simulink model "EchtwertVergleich"  (R2021b)
settings: Solver=VariableStepAuto  StartTime=0.0  StopTime=11  RelTol=1e-3
values from neighbouring files (symbols this model uses):
  T = readtable("YawInertiaPendel01.csv")    [ImportTest.m]
settings Model: Creator=tim  LastModifiedBy=tim

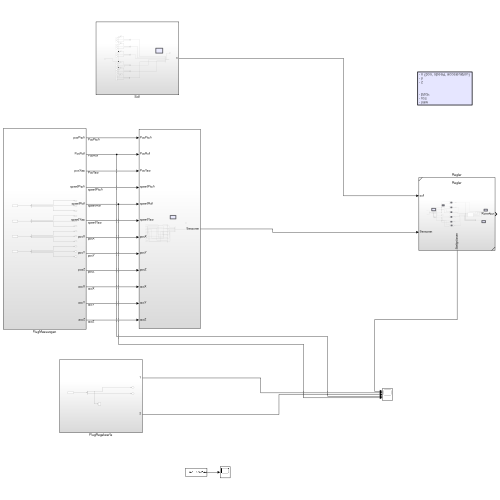
[thumbnail: Simulink's stored preview of the top-level diagram]
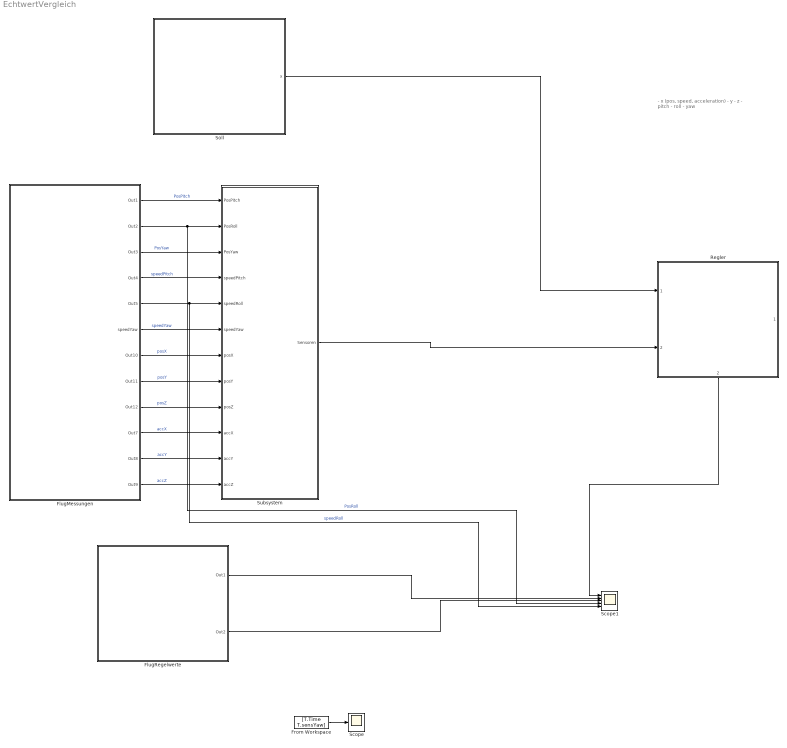
== system EchtwertVergleich ==
  note: - x (pos, speed, acceleration)
      | - y
      | - z
      |
      |
      | - pitch
      | - roll
      | - yaw
  FlugMessungen : Subsystem
  FlugRegelwerte : Subsystem
  From Workspace : FromWorkspace  VariableName=[T.Time T.sensYaw]  SampleTime=T.Time(2) - T.Time(1)  ZeroCross=off  OutputAfterFinalValue=Holding final value
  Regler : Subsystem  VariantControl=Choice  ReferencedSubsystem=Regler
      settings: PortSchema="{\"entries\":[{\"content\":{\"sides\":[{\"content\":{\"connectorIds\":[\"In1\",\"In2\"]},\"type\":\"ConnectorPlacement.EquallySpacedRectSide\",\"uuid\":\"5555f1c3-3fce-4abf-9ec7-ee9d2aa201b7\"},{\"content\":{\"connectorIds\":[\"Out1\"],\"side\":\"RIGHT\"},\"type\":\"ConnectorPlacement.EquallySpacedRectSide\",\"uuid\":\"426c5255-79a7-46e4-b0a4-b934f06d6de9\"},{\"content\":{\"connectorIds\":[],\"side\":\"TOP\"},\"type\":\"ConnectorPlacement.EquallySpacedRectSide\",\"uuid\":\"d67f9dd2-7469-42d8-a750-e83b535a436f\"},{\"content\":{\"connectorIds\":[\"Out2\"],\"side\":\"BOTTOM\"},\"type\":\"ConnectorPlacement.EquallySpacedRectSide\",\"uuid\":\"7dee37cc-875e-40cb-80e0-9d0af31dfaad\"}]},\"type\":\"ConnectorPlacement.EquallySpacedConnector\",\"uuid\":\"ab5c7b53-c15f-43f7-a95d-050bca66474b\"}],\"packageUris\":[\"http://schema.mathworks.com/mf0/Connector/R2020b\"],\"version\":\"1.0\"}"
  Scope : Scope
  Scope1 : Scope  NumInputPorts=5
  Soll : Subsystem
  Subsystem : Subsystem
  wires:
  Soll/1(x) -> Regler/1
  FlugMessungen/1(Out1) -> Subsystem/1(PosPitch)  "PosPitch"
  FlugMessungen/2(Out2) -> Scope1/4, Subsystem/2(PosRoll)  "PosRoll"
  FlugMessungen/3(Out3) -> Subsystem/3(PosYaw)  "PosYaw"
  FlugMessungen/4(Out4) -> Subsystem/4(speedPitch)  "speedPitch"
  FlugMessungen/5(Out5) -> Scope1/5, Subsystem/5(speedRoll)  "speedRoll"
  FlugMessungen/6(speedYaw) -> Subsystem/6(speedYaw)  "speedYaw"
  FlugMessungen/7(Out10) -> Subsystem/7(posX)  "posX"
  FlugMessungen/8(Out11) -> Subsystem/8(posY)  "posY"
  FlugMessungen/9(Out12) -> Subsystem/9(posZ)  "posZ"
  FlugMessungen/10(Out7) -> Subsystem/10(accX)  "accX"
  FlugMessungen/11(Out8) -> Subsystem/11(accY)  "accY"
  FlugMessungen/12(Out9) -> Subsystem/12(accZ)  "accZ"
  Subsystem/1(Sensoren) -> Regler/2
  FlugRegelwerte/1(Out1) -> Scope1/2
  FlugRegelwerte/2(Out2) -> Scope1/3
  Regler/2 -> Scope1/1
  From Workspace/1 -> Scope/1

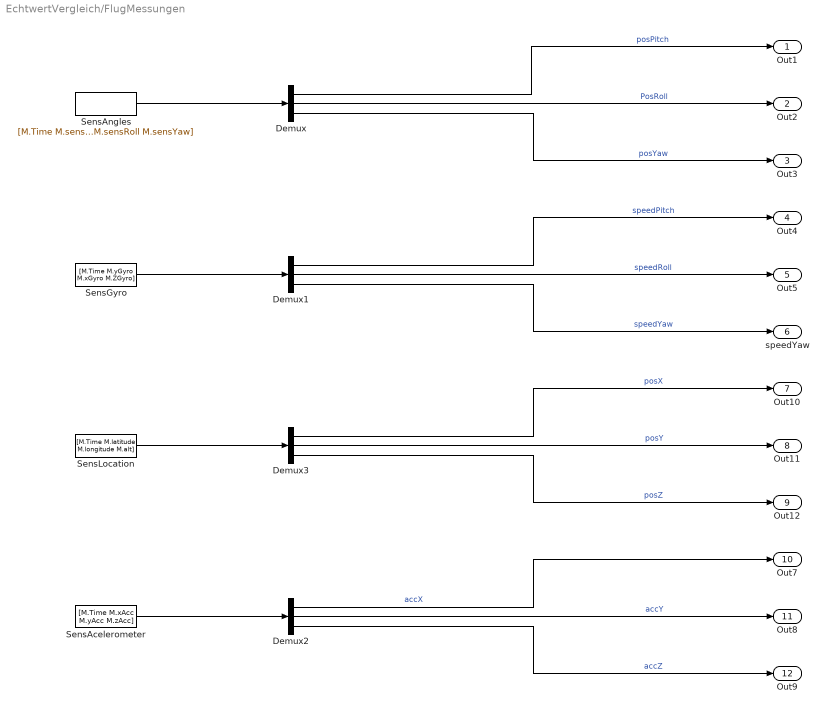
== system EchtwertVergleich/FlugMessungen ==
  Demux{,1..3} (4 alike) : Demux  Outputs=3
  SensAcelerometer : FromWorkspace  VariableName=[M.Time M.xAcc M.yAcc M.zAcc]
  SensAngles : FromWorkspace  VariableName=[M.Time M.sensPitch M.sensRoll M.sensYaw]
  SensGyro : FromWorkspace  VariableName=[M.Time M.yGyro M.xGyro M.ZGyro]
  SensLocation : FromWorkspace  VariableName=[M.Time M.latitude M.longitude M.alt]
  Out1 : Outport
  Out2 : Outport  Port=2
  Out3 : Outport  Port=3
  Out4 : Outport  Port=4
  Out5 : Outport  Port=5
  speedYaw : Outport  Port=6
  Out10 : Outport  Port=7
  Out11 : Outport  Port=8
  Out12 : Outport  Port=9
  Out7 : Outport  Port=10
  Out8 : Outport  Port=11
  Out9 : Outport  Port=12
  wires:
  Demux/1 -> Out1/1  "posPitch"
  Demux/2 -> Out2/1  "PosRoll"
  Demux/3 -> Out3/1  "posYaw"
  Demux1/2 -> Out5/1  "speedRoll"
  Demux2/2 -> Out8/1  "accY"
  Demux2/1 -> Out7/1  "accX"
  Demux2/3 -> Out9/1  "accZ"
  Demux1/3 -> speedYaw/1  "speedYaw"
  Demux1/1 -> Out4/1  "speedPitch"
  Demux3/1 -> Out10/1  "posX"
  Demux3/2 -> Out11/1  "posY"
  Demux3/3 -> Out12/1  "posZ"
  SensAcelerometer/1 -> Demux2/1
  SensLocation/1 -> Demux3/1
  SensAngles/1 -> Demux/1
  SensGyro/1 -> Demux1/1

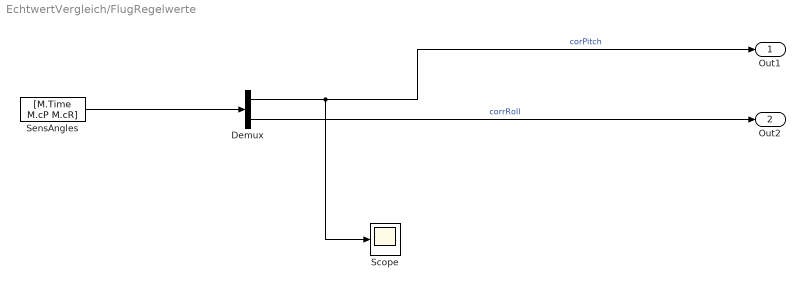
== system EchtwertVergleich/FlugRegelwerte ==
  Demux : Demux  Outputs=2
  Scope : Scope
  SensAngles : FromWorkspace  VariableName=[M.Time M.cP M.cR]  OutputAfterFinalValue=Holding final value
  Out1 : Outport
  Out2 : Outport  Port=2
  wires:
  Demux/2 -> Out2/1  "corrRoll"
  Demux/1 -> Scope/1, Out1/1  "corPitch"
  SensAngles/1 -> Demux/1

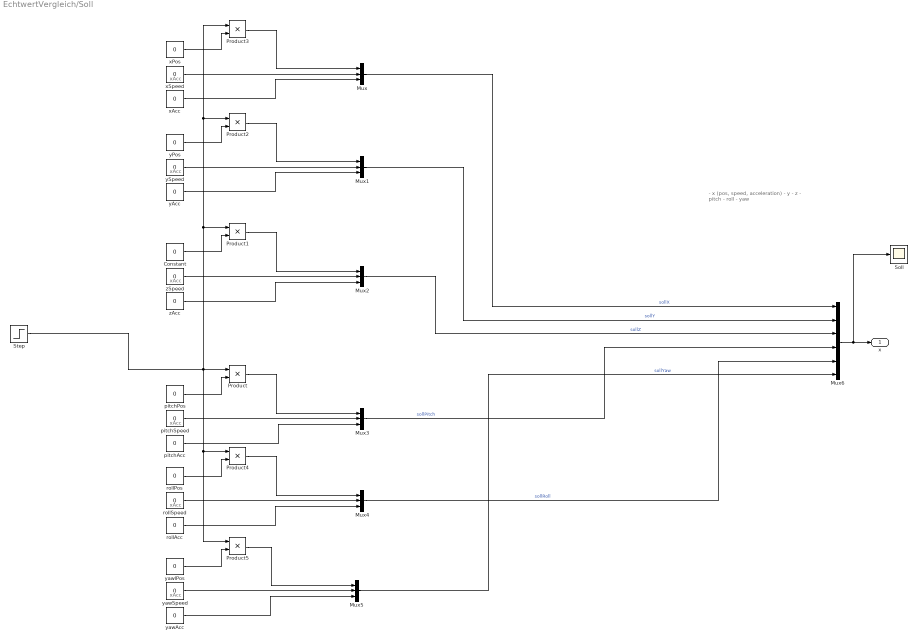
== system EchtwertVergleich/Soll ==
  note: - x (pos, speed, acceleration)
      | - y
      | - z
      |
      |
      | - pitch
      | - roll
      | - yaw
  note: xAcc
  note: xAcc
  note: xAcc
  note: xAcc
  note: xAcc
  note: xAcc
  Constant : Constant  Value=0
  Mux{,1..5} (6 alike) : Mux  Inputs=3
  Mux6 : Mux  Inputs=6
  Product{,1..5} (6 alike) : Product
  Soll : Scope
  Step : Step  SampleTime=0
  pitchAcc : Constant  Value=0
  pitchPos : Constant  Value=0
  pitchSpeed : Constant  Value=0
  rollAcc : Constant  Value=0
  rollPos : Constant  Value=0
  rollSpeed : Constant  Value=0
  xAcc : Constant  Value=0
  xPos : Constant  Value=0
  xSpeed : Constant  Value=0
  yAcc : Constant  Value=0
  yPos : Constant  Value=0
  ySpeed : Constant  Value=0
  yawAcc : Constant  Value=0
  yawSpeed : Constant  Value=0
  yawlPos : Constant  Value=0
  zAcc : Constant  Value=0
  zSpeed : Constant  Value=0
  x : Outport
  wires:
  Mux/1 -> Mux6/1  "sollX"
  Mux1/1 -> Mux6/2  "sollY"
  Mux2/1 -> Mux6/3  "sollZ"
  Mux4/1 -> Mux6/5  "sollRoll"
  Mux5/1 -> Mux6/6  "sollYaw"
  Mux3/1 -> Mux6/4  "sollPitch"
  Mux6/1 -> Soll/1, x/1
  pitchAcc/1 -> Mux3/3
  pitchSpeed/1 -> Mux3/2
  Product/1 -> Mux3/1
  pitchPos/1 -> Product/2
  zAcc/1 -> Mux2/3
  zSpeed/1 -> Mux2/2
  Product1/1 -> Mux2/1
  Constant/1 -> Product1/2
  yAcc/1 -> Mux1/3
  ySpeed/1 -> Mux1/2
  Product2/1 -> Mux1/1
  yPos/1 -> Product2/2
  xAcc/1 -> Mux/3
  xSpeed/1 -> Mux/2
  Product3/1 -> Mux/1
  xPos/1 -> Product3/2
  rollAcc/1 -> Mux4/3
  rollSpeed/1 -> Mux4/2
  Product4/1 -> Mux4/1
  rollPos/1 -> Product4/2
  yawlPos/1 -> Product5/2
  yawSpeed/1 -> Mux5/2
  yawAcc/1 -> Mux5/3
  Product5/1 -> Mux5/1
  Step/1 -> Product3/1, Product2/1, Product1/1, Product5/1, Product4/1, Product/1

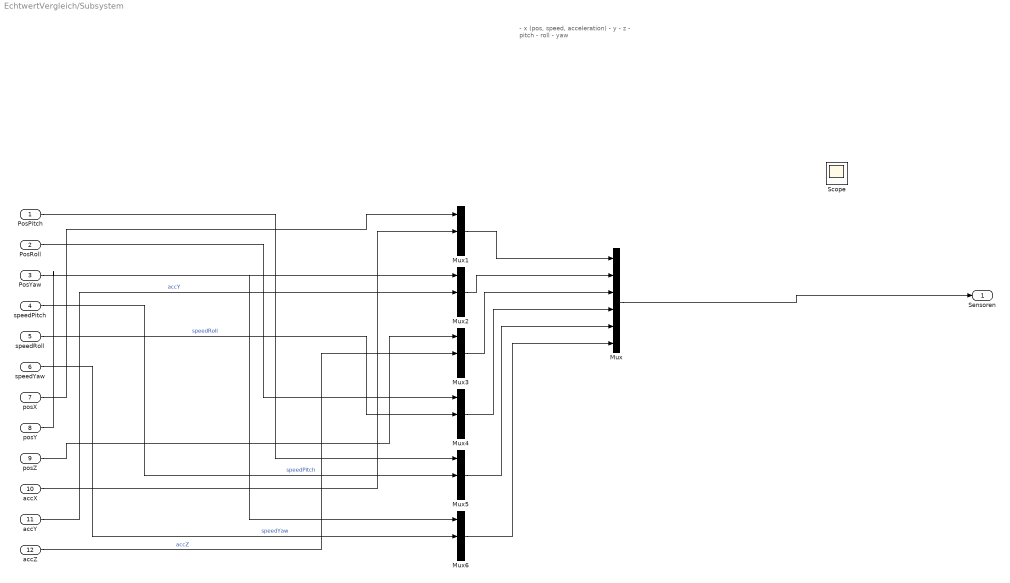
== system EchtwertVergleich/Subsystem ==
  note: - x (pos, speed, acceleration)
      | - y
      | - z
      |
      |
      | - pitch
      | - roll
      | - yaw
  PosPitch : Inport
  PosRoll : Inport  Port=2
  PosYaw : Inport  Port=3
  speedPitch : Inport  Port=4
  speedRoll : Inport  Port=5
  speedYaw : Inport  Port=6
  posX : Inport  Port=7
  posY : Inport  Port=8
  posZ : Inport  Port=9
  accX : Inport  Port=10
  accY : Inport  Port=11
  accZ : Inport  Port=12
  Mux : Mux  Inputs=6
  Mux{1..6} (6 alike) : Mux  Inputs=3
  Scope : Scope
  Sensoren : Outport
  wires:
  Mux1/1 -> Mux/1
  Mux2/1 -> Mux/2
  Mux3/1 -> Mux/3
  PosYaw/1 -> Mux6/1
  PosPitch/1 -> Mux5/1
  PosRoll/1 -> Mux4/1
  speedPitch/1 -> Mux5/2  "speedPitch"
  speedRoll/1 -> Mux4/2  "speedRoll"
  speedYaw/1 -> Mux6/2  "speedYaw"
  posX/1 -> Mux1/1
  posY/1 -> Mux2/1
  posZ/1 -> Mux3/1
  accX/1 -> Mux1/2
  accY/1 -> Mux2/2  "accY"
  accZ/1 -> Mux3/2  "accZ"
  Mux/1 -> Sensoren/1
  Mux4/1 -> Mux/4
  Mux5/1 -> Mux/5
  Mux6/1 -> Mux/6
